simulink model "Boost_Converter_Matlab_simulink_simulation"  (R2015a)
settings: Solver=ode45  StartTime=0.0  StopTime=inf  RelTol=1e-3
libraries: powerlib x9, fl_lib x8, nesl_utility x3, elec_lib x2
settings Model: Creator=DELL  LastModifiedBy=DELL

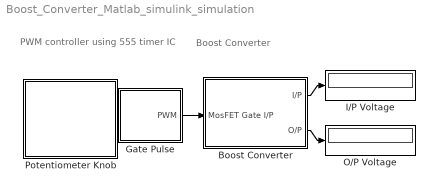
== system Boost_Converter_Matlab_simulink_simulation ==
  note: PWM controller
      | using 555 timer IC
  note: Boost Converter
  Boost Converter : Subsystem
  Gate Pulse : Subsystem
  I/P Voltage : Display
  O/P Voltage : Display
  Potentiometer Knob : Subsystem  DialogController=hmiCreateDDGDialog  IsWebBlock=on  mask(MathWorksWebBlock){webBlockId=d6066df1-86d4-4aee-86bd-51108eb6c511, webBlockType=continuousknob, ShowInLibBrowser=on, ShowInitialText=on, HMISrcModelName=boost_converter}
      mask prompts: webBlockId "WebBlock Id"; webBlockType "WebBlock Type"; HMISrcModelName "Source Model"
      mask Help: helpview([docroot '/mapfiles/simulink.map'], 'hmi_knob')
      mask Display:
      | if strcmp(get_param(bdroot(gcb),'BlockDiagramType'), 'library')
      |     image([(matlabroot) '/toolbox/simulink/hmi/icons/ContinuousKnob.png']);
      | end
  wires:
  Gate Pulse/1(PWM) -> Boost Converter/1(MosFET Gate I/P)
  Boost Converter/1(I/P) -> I/P Voltage/1
  Boost Converter/2(O/P) -> O/P Voltage/1

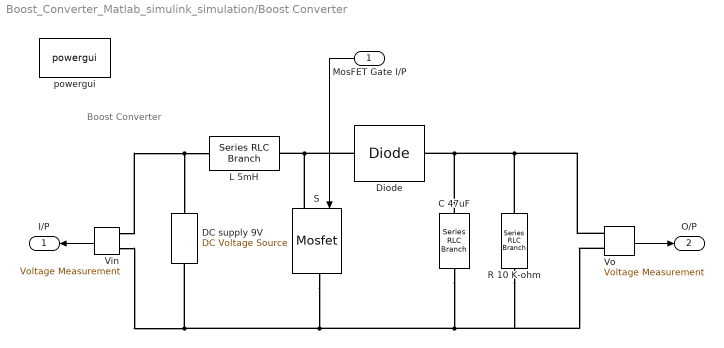
== system Boost_Converter_Matlab_simulink_simulation/Boost Converter ==
  note: Boost Converter
  MosFET Gate I/P : Inport
  C 47uF : powerlib/Elements/Series RLC Branch  LConnTagsString=__new0  RConnTagsString=__new0  BranchType=C  Resistance=1  Inductance=10e-6  SetiL0=off  InitialCurrent=0  Capacitance=47e-6  Setx0=off  InitialVoltage=0  Measurements=None
  DC supply 9V : powerlib/Electrical Sources/DC Voltage Source  Amplitude=9  Measurements=None
  Diode : powerlib/Power Electronics/Diode  Ron=0.001  Lon=0  Vf=0.8  IC=0  UseSnubber=off  Rs=500  Cs=250e-9  Measurements=off
  L 5mH : powerlib/Elements/Series RLC Branch  LConnTagsString=__new0  RConnTagsString=__new0  BranchType=L  Resistance=1  Inductance=5e-3  SetiL0=off  InitialCurrent=0  Capacitance=1e-6  Setx0=off  InitialVoltage=0  Measurements=None
  R 10 K-ohm : powerlib/Elements/Series RLC Branch  LConnTagsString=__new0  RConnTagsString=__new0  BranchType=R  Resistance=10000  Inductance=10e-6  SetiL0=off  InitialCurrent=0  Capacitance=1000e-6  Setx0=off  InitialVoltage=0  Measurements=None
  S : powerlib/Power Electronics/Mosfet  Ron=0.1  Lon=0  Rd=0.01  Vfd=0  IC=0  Rs=1e5  Cs=inf  Measurements=off
  Vin : powerlib/Measurements/Voltage Measurement  PhasorSimulation=off  OutputType=Complex  PSBequivalent=0
  Vo : powerlib/Measurements/Voltage Measurement  PhasorSimulation=off  OutputType=Complex  PSBequivalent=0
  powergui : powerlib/powergui  Priority=1  SimulationMode=Continuous  SolverType=Tustin/Backward Euler (TBE)  SampleTime=10  frequency=60  SPID=off  DisableSnubberDevices=off  DisableRonSwitches=off  DisableVfSwitches=off  SwTol=0  DisplayEquations=off  Interpol=off  methode=off  Ts=100  FunctionMessages=off  echomessages=off  HookPort=off  EnableUseOfTLC=off  x0status=blocks  frequencyindice=0  Pbase=100e6  ErrMax=1e-4  Iterations=50  UnitsV=kV  UnitsW=MW  buscounter=0  RestoreLinks=warning  ResistiveCurrentMeasurement=off  Frange=[0:2:500]  Ylog=off  Xlog=on  ShowGrid=off  save=off  variable=ZData  structure=0  ZoomFFT=off  StartTime=0.0  cycles=1  DisplayStyle=1  fundamental=60  FreqAxis=off  MaxFrequency=1000  frequencyindicesteady=1  RmsSteady=1  display=off
  I/P : Outport
  O/P : Outport  Port=2
  wires:
  Vin/1 -> I/P/1
  MosFET Gate I/P/1 -> S/1
  Vo/1 -> O/P/1
  connections:
  Vin/LConn1 -- DC supply 9V/RConn1 -- L 5mH/LConn1
  Vo/LConn1 -- R 10 K-ohm/LConn1 -- C 47uF/LConn1 -- Diode/RConn1
  C 47uF/RConn1 -- Vo/LConn2 -- R 10 K-ohm/RConn1 -- Vin/LConn2 -- DC supply 9V/LConn1 -- S/RConn1
  Diode/LConn1 -- S/LConn1 -- L 5mH/RConn1

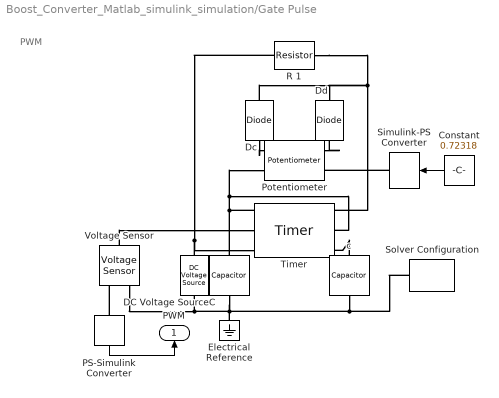
== system Boost_Converter_Matlab_simulink_simulation/Gate Pulse ==
  note: PWM
  C : fl_lib/Electrical/Electrical Elements/Capacitor  c=330e-12 F  r=1e-6 Ohm  g=0 1/Ohm  i_specify=off  i_priority=High  i=0 A  v_specify=off  v_priority=High  v=0 V  vc_specify=off  vc_priority=High  vc=0 V
  Constant : Constant  Value=0.72318
  DC Voltage Source : fl_lib/Electrical/Electrical Sources/DC Voltage Source  v0=20 V
  Dc : fl_lib/Electrical/Electrical Elements/Diode  Vf=0.6 V  Ron=0.3 Ohm  Goff=1e-8 1/Ohm  i_specify=off  i_priority=High  i=0 A  v_specify=off  v_priority=High  v=0 V
  Dd : fl_lib/Electrical/Electrical Elements/Diode  Vf=0.6 V  Ron=0.3 Ohm  Goff=1e-8 1/Ohm  i_specify=off  i_priority=High  i=0 A  v_specify=off  v_priority=High  v=0 V
  Electrical Reference : fl_lib/Electrical/Electrical Elements/Electrical Reference
  PS-Simulink Converter : nesl_utility/PS-Simulink Converter  PhysicalDomain=network_engine_domain  SubClassName=ps_output  LeftPortType=input  RightPortType=output  PseudoPeriodic=off  Frequencies=[]  Unit=1  AffineConversion=off
  Potentiometer : elec_lib/Passive Devices/Potentiometer  R0=47 kOhm  Rw=1 Ohm  Rcenter=200 Ohm  xmin=0  xmax=1  Taper=1  Gradient=1  xminL=0  xmaxL=1  lambda=1  A=1 Ohm
  R 1 : fl_lib/Electrical/Electrical Elements/Resistor  R=10 kOhm  i_specify=off  i_priority=High  i=0 A  v_specify=off  v_priority=High  v=0 V
  Simulink-PS Converter : nesl_utility/Simulink-PS Converter  PhysicalDomain=network_engine_domain  SubClassName=ps_input  LeftPortType=input  RightPortType=output  PseudoPeriodic=off  Frequencies=[]  NoiseDistribution=none  NoiseParameters=[]  Unit=1  AffineConversion=off  InputFiltering=off  SimscapeFilterOrder=1  InputFilterTimeConstant=0.001  UdotUserProvided=1
  Solver Configuration : nesl_utility/Solver Configuration  PhysicalDomain=network_engine_domain  SubClassName=solver  LeftPortType=input  RightPortType=generic  Accelerate=off  Tones=[]  Harmonics=[]  SimulateNoise=off  Profile=off  UseLocalSampling=off  EnableSwitchedLinearOptims=on  FrequencyDomain=off  UseCCode=off  RelTol=0.001  AbsTol=1e-06  MinStep=1e-09  ToWorkspace=off  RevertToSquareIcSolve=off  NumHomotopyIterations=100  DoDC=off  ResidualTolerance=1e-09  UseLocalSolver=off  LocalSolverChoice=NE_BACKWARD_EULER_ADVANCER  LocalSolverSampleTime=0.001  DoFixedCost=off  MaxNonlinIter=3  MaxModeIter=2  LinearAlgebra=Sparse  DelaysMemoryBudget=1024  AutomaticFiltering=on  FilteringTimeConstant=0.001
  Timer : elec_lib/Integrated Circuits/Timer  V_CC=15 V  V_OL=0 V  V_OH=14.1 V  R_OUT=8 Ohm  Delay=1e-7 s  R_DIV=5 kOhm  R_closed=12 Ohm  R_open=5e+8 Ohm
  Voltage Sensor : fl_lib/Electrical/Electrical Sensors/Voltage Sensor
  c : fl_lib/Electrical/Electrical Elements/Capacitor  c=330e-12 F  r=1e-6 Ohm  g=0 1/Ohm  i_specify=off  i_priority=High  i=0 A  v_specify=off  v_priority=High  v=0 V  vc_specify=off  vc_priority=High  vc=0 V
  PWM : Outport
  wires:
  PS-Simulink Converter/1 -> PWM/1
  Constant/1 -> Simulink-PS Converter/1
  connections:
  R 1/RConn1 -- Dc/LConn1 -- Dd/RConn1 -- Timer/RConn1
  Simulink-PS Converter/RConn1 -- Potentiometer/RConn2
  PS-Simulink Converter/LConn1 -- Voltage Sensor/RConn1
  c/LConn1 -- Timer/RConn3
  C/LConn1 -- Timer/LConn1 -- Timer/RConn2 -- Potentiometer/LConn2
  DC Voltage Source/LConn1 -- R 1/LConn1 -- Timer/LConn3
  Dc/RConn1 -- Potentiometer/LConn1
  c/RConn1 -- Solver Configuration/RConn1 -- Electrical Reference/LConn1 -- C/RConn1 -- Voltage Sensor/RConn2 -- DC Voltage Source/RConn1
  Voltage Sensor/LConn1 -- Timer/LConn2
  Potentiometer/RConn1 -- Dd/LConn1

== system Boost_Converter_Matlab_simulink_simulation/Potentiometer Knob ==
